simulink model "Model"  (R2024b)
settings: Solver=ode45  StartTime=0.0  StopTime=10.0  RelTol=1e-3
InitFcn:
  | Main
values from neighbouring files (symbols this model uses):
  A = [0, 1; -2 -40]    [Main.m]
  Ao = Ad - L * Cd    [Main.m]
  B = [0; 40]    [Main.m]
  Bo = [Bd, L]    [Main.m]
  C = [1, 0]    [Main.m]
  Co = eye(2)    [Main.m]
  D = 0    [Main.m]
  Do = zeros(2)    [Main.m]
  K = K(2:3)    [Main.m]
  Nr = Nu + K * Nx    [Main.m]
  Ts = 0.01    [Main.m]
undefined symbols (not defined in the file or in its folder): DiscIntNeverNeededParam
settings Model: Creator=Banaan  LastModifiedBy=Banaan

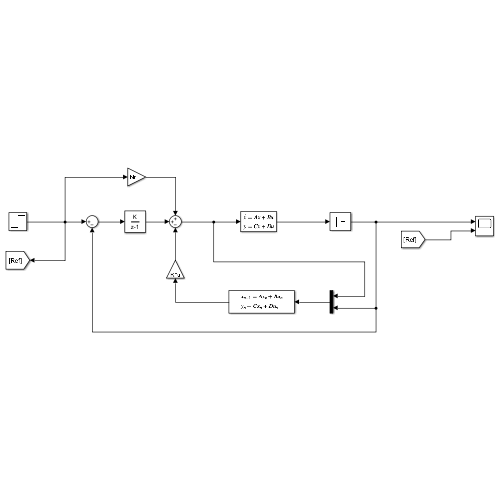
[thumbnail: Simulink's stored preview of the top-level diagram]
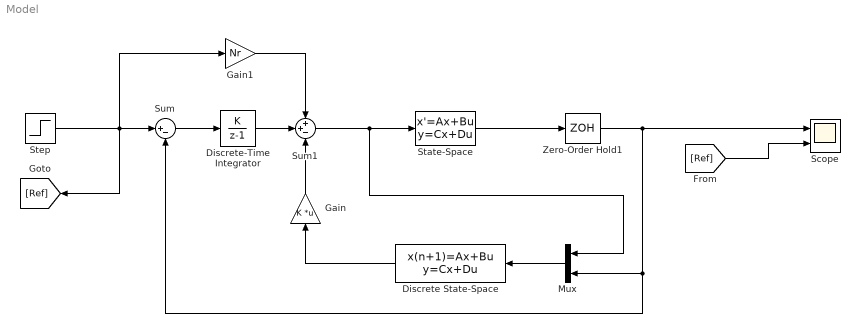
== system Model ==
  Discrete State-Space : DiscreteStateSpace  A=Ao  B=Bo  C=Co  D=Do  SampleTime=Ts
  Discrete-Time Integrator : DiscreteIntegrator  IntegratorMethod=Accumulation: Forward Euler  gainval=Ki  SampleTime=Ts  ICPrevOutput=DiscIntNeverNeededParam  ICPrevScaledInput=DiscIntNeverNeededParam
  Gain : Gain  Gain=K  Multiplication=Matrix(K*u)
  Gain1 : Gain  Gain=Nr
  Mux : Mux  Inputs=2
  Scope : Scope  NumInputPorts=2
  State-Space : StateSpace  A=A  B=B  C=C  D=D  InitialCondition=0
  Step : Step  SampleTime=0
  Sum : Sum  Inputs=|+-
  Sum1 : Sum  Inputs=++-
  Zero-Order Hold1 : ZeroOrderHold  SampleTime=Ts
  wires:
  Sum1/1 -> State-Space/1, Mux/1
  Zero-Order Hold1/1 -> Scope/1, Sum/2, Mux/2
  Sum/1 -> Discrete-Time Integrator/1
  Gain/1 -> Sum1/3
  Discrete State-Space/1 -> Gain/1
  Mux/1 -> Discrete State-Space/1
  State-Space/1 -> Zero-Order Hold1/1
  Discrete-Time Integrator/1 -> Sum1/2
  Gain1/1 -> Sum1/1
  Step/1 -> [Ref], Gain1/1, Sum/1
  [Ref] -> Scope/2
